simulink model "vel_est_test"  (R2024b)
settings: Solver=VariableStepAuto  StartTime=0.0  StopTime=200  RelTol=1e-3
values from neighbouring files (symbols this model uses):
  str = resampleStruct(dat_fixed, dat_fixed, 0:0.01:200)    [ekf_test.m]
settings Model: Creator=rcmas  LastModifiedBy=rcmas

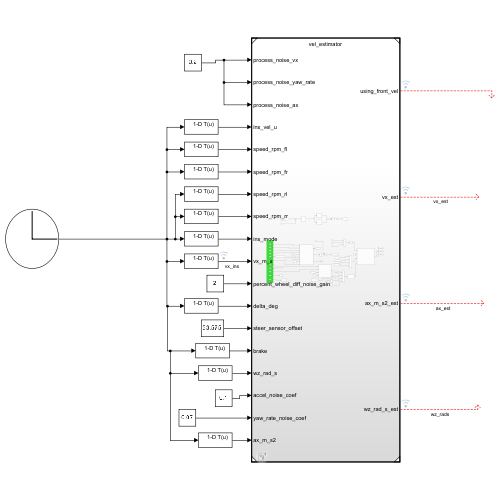
[thumbnail: Simulink's stored preview of the top-level diagram]
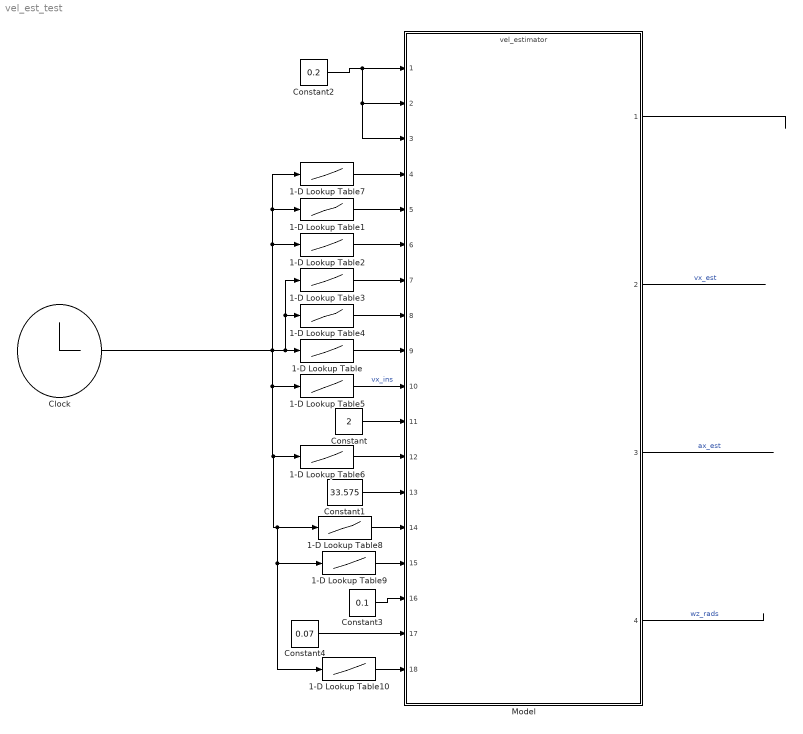
== system vel_est_test ==
  1-D Lookup Table : Lookup_n-D  NumberOfTableDimensions=1  BreakpointsForDimension1=str.globalTime  Table=str.VNData.status.ins_mode_int  InternalRulePriority=Speed  RndMeth=Simplest
  1-D Lookup Table1 : Lookup_n-D  NumberOfTableDimensions=1  BreakpointsForDimension1=str.globalTime  Table=str.inv1_dynamics.actual_speed_rpm  InternalRulePriority=Speed  RndMeth=Simplest
  1-D Lookup Table10 : Lookup_n-D  NumberOfTableDimensions=1  BreakpointsForDimension1=str.globalTime  Table=str.VNData.vn_linear_accel_m_ss.x  InternalRulePriority=Speed  RndMeth=Simplest
  1-D Lookup Table2 : Lookup_n-D  NumberOfTableDimensions=1  BreakpointsForDimension1=str.globalTime  Table=str.inv2_dynamics.actual_speed_rpm  InternalRulePriority=Speed  RndMeth=Simplest
  1-D Lookup Table3 : Lookup_n-D  NumberOfTableDimensions=1  BreakpointsForDimension1=str.globalTime  Table=str.inv3_dynamics.actual_speed_rpm  InternalRulePriority=Speed  RndMeth=Simplest
  1-D Lookup Table4 : Lookup_n-D  NumberOfTableDimensions=1  BreakpointsForDimension1=str.globalTime  Table=str.inv4_dynamics.actual_speed_rpm  InternalRulePriority=Speed  RndMeth=Simplest
  1-D Lookup Table5 : Lookup_n-D  NumberOfTableDimensions=1  BreakpointsForDimension1=str.globalTime  Table=str.VNData.vn_vel_m_s.x  InternalRulePriority=Speed  RndMeth=Simplest
  1-D Lookup Table6 : Lookup_n-D  NumberOfTableDimensions=1  BreakpointsForDimension1=str.globalTime  Table=str.steering_data.steering_analog_raw  InternalRulePriority=Speed  RndMeth=Simplest
  1-D Lookup Table7 : Lookup_n-D  NumberOfTableDimensions=1  BreakpointsForDimension1=str.globalTime  Table=str.VNData.status.ins_vel_u  InternalRulePriority=Speed  RndMeth=Simplest
  1-D Lookup Table8 : Lookup_n-D  NumberOfTableDimensions=1  BreakpointsForDimension1=str.globalTime  Table=str.pedals_system_data.brake_pedal  InternalRulePriority=Speed  RndMeth=Simplest
  1-D Lookup Table9 : Lookup_n-D  NumberOfTableDimensions=1  BreakpointsForDimension1=str.globalTime  Table=str.VNData.vn_angular_rate_rad_s.z  InternalRulePriority=Speed  RndMeth=Simplest
  Clock : Clock
  Constant : Constant  Value=2
  Constant1 : Constant  Value=33.575
  Constant2 : Constant  Value=0.2
  Constant3 : Constant  Value=0.1
  Constant4 : Constant  Value=0.07
  Model : ModelReference  ModelNameDialog=vel_estimator.slx  SimulationMode=Normal  ModelReferenceVersion=1.40
  wires:
  1-D Lookup Table/1 -> Model/9
  Clock/1 -> 1-D Lookup Table5/1, 1-D Lookup Table10/1, 1-D Lookup Table9/1, 1-D Lookup Table8/1, 1-D Lookup Table6/1, 1-D Lookup Table4/1, 1-D Lookup Table3/1, 1-D Lookup Table/1, 1-D Lookup Table2/1, 1-D Lookup Table7/1, 1-D Lookup Table1/1
  1-D Lookup Table1/1 -> Model/5
  1-D Lookup Table2/1 -> Model/6
  1-D Lookup Table3/1 -> Model/7
  1-D Lookup Table4/1 -> Model/8
  1-D Lookup Table5/1 -> Model/10  "vx_ins"
  Constant/1 -> Model/11
  1-D Lookup Table6/1 -> Model/12
  Constant1/1 -> Model/13
  1-D Lookup Table7/1 -> Model/4
  Constant2/1 -> Model/3, Model/2, Model/1
  1-D Lookup Table8/1 -> Model/14
  1-D Lookup Table9/1 -> Model/15
  1-D Lookup Table10/1 -> Model/18
  Constant3/1 -> Model/16
  Constant4/1 -> Model/17
  Model/1 -> ?
  Model/2 -> ?  "vx_est"
  Model/3 -> ?  "ax_est"
  Model/4 -> ?  "wz_rads"
